simulink model "Sim_Model_2ndODE_ex3"  (Simulink 8.0)
settings: Solver=ode45  StartTime=0.0  StopTime=10.0  RelTol=1e-3
settings Model: Creator=David  LastModifiedBy=David
settings DataIOCC: SignalLoggingSaveFormat=ModelDataLogs
settings DebuggingCC: FcnCallInpInsideContextMsg=UseLocalSettings
settings GRTTargetCC: CombineOutputUpdateFcns=off  GRTInterface=on

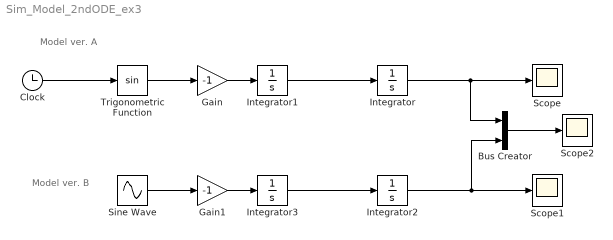
== system Sim_Model_2ndODE_ex3 ==
  note: Model ver. B
  note: Model ver. A
  Bus Creator : BusCreator  Inputs=2
  Clock : Clock
  Gain : Gain  Gain=-1
  Gain1 : Gain  Gain=-1
  Integrator{,1..3} (4 alike) : Integrator
  Scope : Scope
  Scope1 : Scope
  Scope2 : Scope
      settings: SaveName=ScopeData2
  Sine Wave : Sin  SampleTime=0
  Trigonometric Function : Trigonometry
  wires:
  Integrator1/1 -> Integrator/1
  Integrator/1 -> Bus Creator/1, Scope/1
  Clock/1 -> Trigonometric Function/1
  Trigonometric Function/1 -> Gain/1
  Gain/1 -> Integrator1/1
  Integrator3/1 -> Integrator2/1
  Integrator2/1 -> Bus Creator/2, Scope1/1
  Sine Wave/1 -> Gain1/1
  Gain1/1 -> Integrator3/1
  Bus Creator/1 -> Scope2/1
